simulink library "filteredPDController_ul"  (R2018b)
settings: Solver=VariableStepAuto  StartTime=0.0  StopTime=10.0  RelTol=1e-3
settings Model: Creator=mcobb  LastModifiedBy=mae-ncsucore

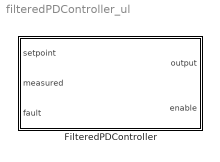
== system filteredPDController_ul ==
  FilteredPDController : Subsystem  mask{enable=off, kp=1, kd=0, timeConstant_s=0.1, intialError=0, initialOutput=0}
      mask prompts: kp "Proportional Gain"; kd "Derivative Gain"; timeConstant_s "Time Constant [s]"; intialError "Initial Error"; initialOutput "Initial Output"
      mask TypeOptions kp: kp/Value
      mask TypeOptions kd: kd/Value
      mask TypeOptions timeConstant_s: timeConstant_s/Value
      mask DialogControl Control3 Prompt: Gains & Time Constants
      mask DialogControl Control2 Prompt: Initial Conditions
      mask Display:
      | port_label('input',1,'Setpoint')
      | port_label('input',2,'Measured')
      | port_label('input',3,'Fault')
      | 
      | port_label('output',1,'Command')
      | 
      | enbl = get_param(gcb,'enable');
      | 
      | if strcmpi(enbl,'on')
      |     color = [0 0.7 0];
      |     str = 'ENABLED';
      | else
      |     color = [0.7 0 0];
      |     str = 'DISABLED';
      | end
      | patch([0 1 1 0], [0.9 0.9 1 1],color)
      | 
      | str_kp = get_param(gcb,'kp');
      | str_kd = get_param(gcb,'kd');
      | str_timeC = get_param(gcb,'timeConstant_s');
      | 
      | if contains(str_kp,'Value')
      |     dict = Simulink.data.dictionary.open('paramsDataDictionary.sldd');
      |     sect = getSection(dict,'Design Data');
      |     str_n = strsplit(str_kp,'.');
      |     var = getEntry(sect,str_n{1});
      |     val = getValue(var);
      |     str_kp = num2str(val.Value);
      |     str = [str '\newline {\fontname{Cambria Math}K_p = ' str_kp];
      | 
      |     str_n = strsplit(str_kd,'.');
      |     var = getEntry(sect,str_n{1});
      |     val = getValue(var);
      |     str_kd = num2str(val.Value);
      |     str = [str '\newline K_d = ' str_kd ];
      | 
      |     str_n = strsplit(str_timeC,'.');
      |     var = getEntry(sect,str_n{1});
      |     val = getValue(var);
      |     str_timeC = num2str(val.Value);
      |     str = [str '\newline \tau   = ' str_timeC '}'];
      | else
      |     str = [str '\newline {\fontname{Cambria Math}K_p = ' str_kp];
      |     str = [str '\newline K_d = ' str_kd];
      |     str = [str '\newline \tau   = ' str_timeC '}'];
      | end
      | 
      | disp(str,'texmode','on')

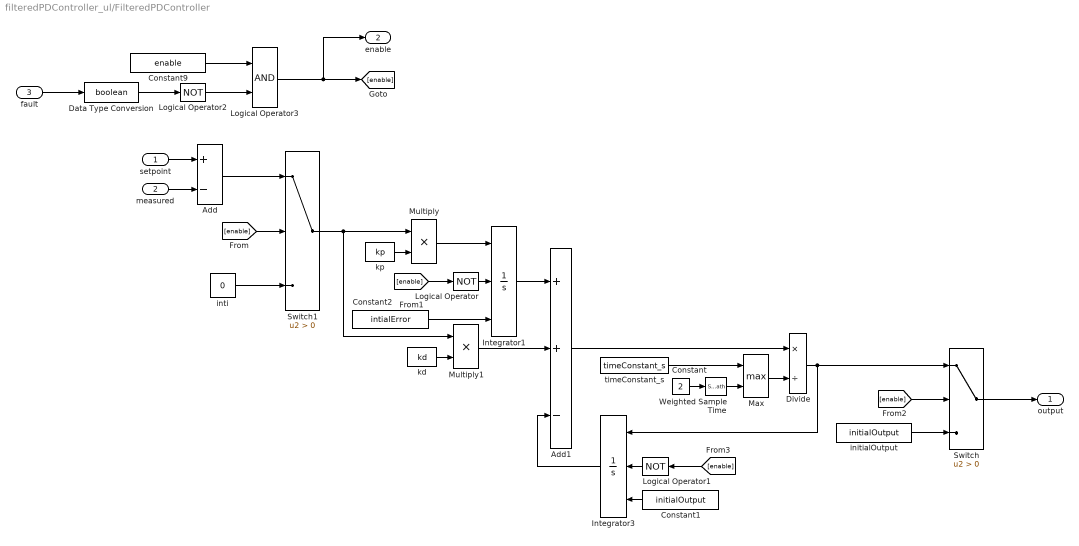
== system filteredPDController_ul/FilteredPDController ==
  setpoint : Inport
  measured : Inport  Port=2
  fault : Inport  Port=3
  Add : Sum  Inputs=+-
  Add1 : Sum  Inputs=++-
  Constant : Constant  Value=2
  Constant1 : Constant  Value=initialOutput
  Constant2 : Constant  Value=intialError
  Constant9 : Constant  Value=enable
  Data Type Conversion : DataTypeConversion  OutDataTypeStr=boolean
  Divide : Product  Inputs=*/
  Integrator1 : Integrator  ExternalReset=rising  InitialConditionSource=external  InitialCondition=0.001
  Integrator3 : Integrator  ExternalReset=level  InitialConditionSource=external  InitialCondition=0.001
  Logical Operator : Logic  Operator=NOT  AllPortsSameDT=off  OutDataTypeStr=boolean
  Logical Operator1 : Logic  Operator=NOT  AllPortsSameDT=off  OutDataTypeStr=boolean
  Logical Operator2 : Logic  Operator=NOT  AllPortsSameDT=off  OutDataTypeStr=boolean
  Logical Operator3 : Logic  AllPortsSameDT=off  OutDataTypeStr=boolean
  Max : MinMax  Function=max  Inputs=2
  Multiply : Product
  Multiply1 : Product
  Switch : Switch  Criteria=u2 > Threshold
  Switch1 : Switch  Criteria=u2 > Threshold
  Weighted Sample Time : SampleTimeMath  TsampMathOp=Ts Only  weightValue=1
  initialOutput : Constant  Value=initialOutput
  inti : Constant  Value=0
  kd : Constant  Value=kd
  kp : Constant  Value=kp
  timeConstant_s : Constant  Value=timeConstant_s
  output : Outport
  enable : Outport  Port=2
  wires:
  setpoint/1 -> Add/1
  measured/1 -> Add/2
  timeConstant_s/1 -> Max/1
  Divide/1 -> Switch/1, Integrator3/1
  Weighted Sample Time/1 -> Max/2
  Constant/1 -> Weighted Sample Time/1
  Max/1 -> Divide/2
  Constant1/1 -> Integrator3/3
  Constant2/1 -> Integrator1/3
  Multiply/1 -> Integrator1/1
  kp/1 -> Multiply/2
  kd/1 -> Multiply1/2
  Switch1/1 -> Multiply1/1, Multiply/1
  Integrator1/1 -> Add1/1
  Multiply1/1 -> Add1/2
  Integrator3/1 -> Add1/3
  Add1/1 -> Divide/1
  Logical Operator/1 -> Integrator1/2
  Logical Operator1/1 -> Integrator3/2
  Switch/1 -> output/1
  initialOutput/1 -> Switch/3
  inti/1 -> Switch1/3
  Add/1 -> Switch1/1
  [enable] -> Switch1/2
  [enable] -> Logical Operator/1
  [enable] -> Switch/2
  fault/1 -> Data Type Conversion/1
  Logical Operator2/1 -> Logical Operator3/2
  Logical Operator3/1 -> enable/1, [enable]
  Constant9/1 -> Logical Operator3/1
  [enable] -> Logical Operator1/1
  Data Type Conversion/1 -> Logical Operator2/1
